simulink model "sefdmConv"  (R2022a)
settings: Solver=VariableStepDiscrete  StartTime=0.0  StopTime=infoBitsPerFrame*100  RelTol=1e-3
InitFcn:
  | run('initSefdmModel.m')
StopFcn:
  | % disp(['ber = ', num2str(out.ber(1))]);
values from neighbouring files (symbols this model uses):
  bitAlloc = ones(N1, 1) * bitsPerSymbol    [initSefdmModel.m]
  bitsPerFrame = dataNum * N1 * bitsPerSymbol    (= 16256)    [initSefdmModel.m]
  codeRate = 1/2    (= 0.5)    [initSefdmModel.m]
  dataNum = 16    [initSefdmModel.m]
  fecLength = 32 / parallelFactor    (= 64)    [initSefdmModel.m]
  fftSize = 512    [initSefdmModel.m]
  infoBitsPerFrame = bitsPerFrame * codeRate - parallel * (constLen - 1)    (= 7366)    [initSefdmModel.m]
  intrlvCol = 1    [initSefdmModel.m]
  intrlvRow = parallel * 2    (= 254)    [initSefdmModel.m]
  N1 = 254    [initSefdmModel.m]
  preamble = preamble(channelInUse, :)    [initSefdmModel.m]
  seed = 42    [initSefdmModel.m]
  symbolsPerFrame = bitsPerFrame / bitsPerSymbol    (= 4064)    [initSefdmModel.m]
  useEqualizer = 1    [initSefdmModel.m]
  useInterleave = 1    [initSefdmModel.m]
  useIteration = 0    [initSefdmModel.m]
libraries: commsink2 x2, dspstat3 x2, commrandsrc3 x1, commchan3 x1, dspindex x1
settings Model: Creator=lsfan  LastModifiedBy=lsfan
settings SolverCC: AlgebraicLoopSolver=TrustRegion
settings DataIOCC: LimitDataPoints=on  SaveOutput=off  SaveTime=off
settings OptimizationCC: BooleanDataType=off  DefaultParameterBehavior=Inlined  LocalBlockOutputs=off  LifeSpan=inf
settings DebuggingCC: AlgebraicLoopMsg=error  SingleTaskRateTransMsg=error  UnconnectedInputMsg=warning  UnconnectedOutputMsg=warning  UnconnectedLineMsg=warning  AllowSymbolicDim=off  SFUnexpectedBacktrackingDiag=warning  SFNoUnconditionalDefaultTransitionDiag=warning  SFExecutionAtInitializationDiag=none  SFMachineParentedDataDiag=warning  ArithmeticOperatorsInVariantConditions=warning
settings SFSimCC: SimUseLocalCustomCode=off  CustomCodeUndefinedFunction=UseInterfaceOnly
settings RTWCC: RTWUseLocalCustomCode=off
settings CodeAppCC: StateflowObjectComments=on
settings GRTTargetCC: TargetLangStandard=C89/C90 (ANSI)
settings ConfigComp: CovMetricSettings=dw  CovSaveCumulativeToWorkspaceVar=on  CovSaveSingleToWorkspaceVar=on  CovExternalEMLEnable=off  CovSFcnEnable=off

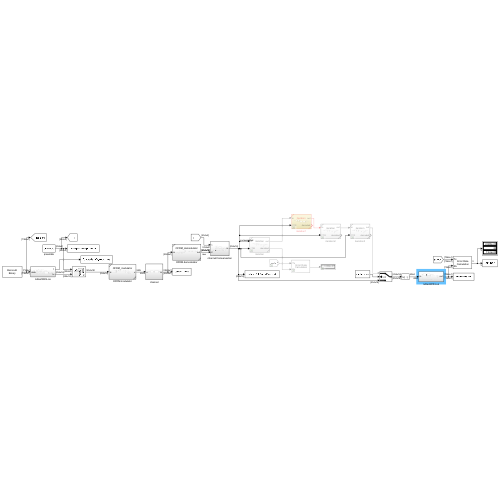
[thumbnail: Simulink's stored preview of the top-level diagram]
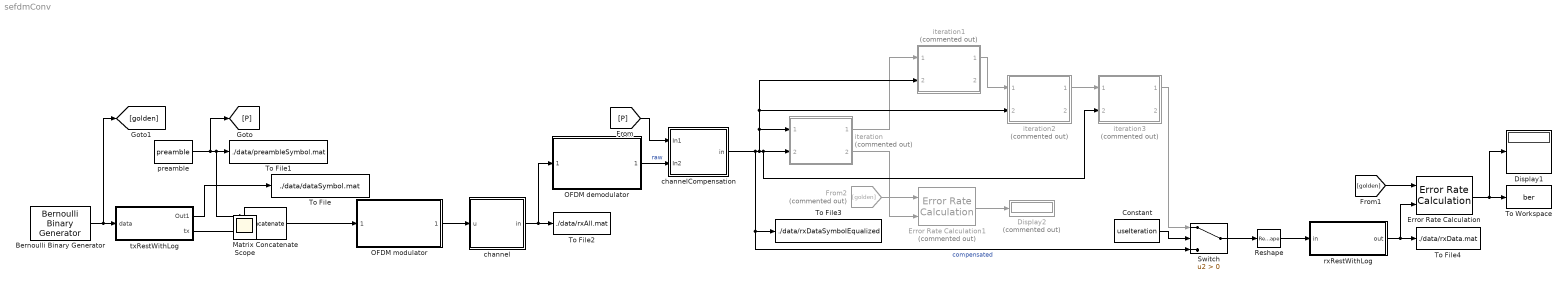
== system sefdmConv ==
  Bernoulli Binary Generator : commrandsrc3/Bernoulli Binary Generator  ProbabilityOfZero=0.5  SeedSource=Parameter  Seed=seed  SampleTime=1  SamplesPerFrame=infoBitsPerFrame  OutputDataType=double  SimulateUsing=Interpreted execution
  Constant : Constant  Value=useIteration
  Display1 : Display
  Display2 : Display  Commented=on
  Error Rate Calculation : commsink2/Error Rate Calculation  N=0  st_delay=0  cp_mode=Entire frame  subframe=[]  PMode=Port  WsName=ErrorVec  RsMode2=off  stop=off  numErr=maxErrNum  maxBits=maxBitsNum
  Error Rate Calculation1 : commsink2/Error Rate Calculation  Commented=on  N=0  st_delay=0  cp_mode=Entire frame  subframe=[]  PMode=Port  WsName=ErrorVec  RsMode2=off  stop=off  numErr=maxErrNum  maxBits=maxBitsNum
  From2 : From  Commented=on  GotoTag=golden
  Matrix Concatenate : Concatenate  Mode=Multidimensional array  ConcatenateDimension=2
  OFDM demodulator : Subsystem  ReferencedSubsystem=OFDM_demodulator
  OFDM modulator : Subsystem  ReferencedSubsystem=OFDM_modulator
  Reshape : Reshape
  Switch : Switch  Criteria=u2 > Threshold  SaturateOnIntegerOverflow=off  InputSameDT=off
  To File : ToFile  Filename=./data/dataSymbol.mat  SaveFormat=Timeseries
  To File1 : ToFile  Filename=./data/preambleSymbol.mat  SaveFormat=Timeseries
  To File2 : ToFile  Filename=./data/rxAll.mat  SaveFormat=Timeseries
  To File3 : ToFile  Filename=./data/rxDataSymbolEqualized  SaveFormat=Timeseries
  To File4 : ToFile  Filename=./data/rxData.mat  SaveFormat=Timeseries
  To Workspace : ToWorkspace  VariableName=ber  SampleTime=-1
      settings: Save2DSignal=2-D array (concatenate along first dimension)
  channel : Subsystem
  channelCompensation : Subsystem
  iteration{,1..3} (4 alike) : Subsystem  Commented=on  ReferencedSubsystem=iteration
  preamble : Constant  Value=preamble
  rxRestWithLog : Subsystem
  txRestWithLog : Subsystem
  Scope : Scope
  wires:
  [golden] -> Error Rate Calculation/1
  iteration2/1 -> iteration3/1
  txRestWithLog/1(Out1) -> To File/1
  txRestWithLog/2(tx) -> Matrix Concatenate/2
  Constant/1 -> Switch/2
  preamble/1 -> Matrix Concatenate/1, To File1/1, [P]
  iteration/1 -> iteration1/1
  From2/1 -> Error Rate Calculation1/1
  OFDM demodulator/1 -> channelCompensation/2(In2)  "raw"
  OFDM modulator/1 -> channel/1(u)
  iteration1/1 -> iteration2/1
  Switch/1 -> Reshape/1
  [P] -> channelCompensation/1(In1)
  Matrix Concatenate/1 -> OFDM modulator/1
  Reshape/1 -> rxRestWithLog/1(in)
  Error Rate Calculation1/1 -> Display2/1
  Bernoulli Binary Generator/1 -> txRestWithLog/1(data), [golden]
  iteration3/1 -> Switch/1
  iteration/2 -> Error Rate Calculation1/2
  Error Rate Calculation/1 -> To Workspace/1, Display1/1
  channel/1(in) -> OFDM demodulator/1, To File2/1
  rxRestWithLog/1(out) -> To File4/1, Error Rate Calculation/2
  channelCompensation/1(in) -> To File3/1, Switch/3, iteration3/2, iteration/2, iteration1/2, iteration2/2, iteration/1  "compensated"

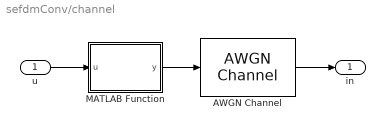
== system sefdmConv/channel ==
  u : Inport
  AWGN Channel : commchan3/AWGN Channel  InputProcessing=Columns as channels (frame based)  seed=67  noiseMode="Signal to noise ratio  (SNR)"  EbNodB=EbNo  EsNodB=10  SNRdB=EbNo  bitsPerSym=bitsPerSymbol  Ps=1 / fftSize  Tsym=bitsPerSymbol  variance=1
  MATLAB Function : MATLAB Function  TreatAsAtomicUnit=on
  in : Outport
  wires:
  MATLAB Function/1(y) -> AWGN Channel/1
  u/1 -> MATLAB Function/1(u)
  AWGN Channel/1 -> in/1

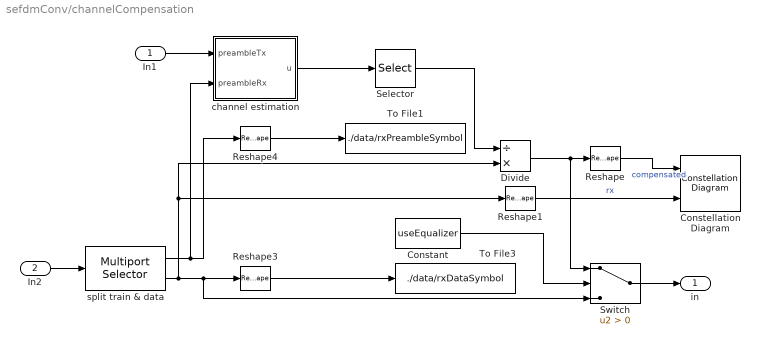
== system sefdmConv/channelCompensation ==
  In1 : Inport
  In2 : Inport  Port=2
  Constant : Constant  Value=useEqualizer
  Constellation Diagram : ConstellationDiagram  NumInputPorts=2  WindowPosition=[2983.000000,244.000000,600.000000,600.000000,]  Visible=on  ScopeFrameLocation=window  ReferenceConstellation="{[16-QAM][0.7071+0.7071i          -0.7071+0.7071i          -0.7071-0.7071i            0.707-0.7071i]}"  ShowLegend=on  DefaultConfigurationName=comm.scopes.ConstellationDiagramBlockCfg
  Divide : Product  Inputs=/*
  Reshape{,1,3..4} (4 alike) : Reshape
  Selector : Selector  NumberOfDimensions=2  InputPortWidth=3  IndexOptions=Select all,Index vector (dialog)  Indices=[1 3],ones(1,dataNum)  OutputSizes=1,1
  Switch : Switch  Criteria=u2 > Threshold  SaturateOnIntegerOverflow=off  InputSameDT=off
  To File1 : ToFile  Filename=./data/rxPreambleSymbol  SaveFormat=Timeseries
  To File3 : ToFile  Filename=./data/rxDataSymbol  SaveFormat=Timeseries
  channel estimation : Subsystem
  split train & data : dspindex/Multiport Selector  rowsOrCols=Columns  idxCellArray={[1:preambleNum], [preambleNum+1:frameNum]}  idxErrMode=Clip Index
  in : Outport
  wires:
  In2/1 -> split train & data/1
  Reshape3/1 -> To File3/1
  Reshape4/1 -> To File1/1
  In1/1 -> channel estimation/1(preambleTx)
  Selector/1 -> Divide/1
  Reshape1/1 -> Constellation Diagram/2  "rx"
  channel estimation/1(u) -> Selector/1
  Constant/1 -> Switch/2
  Switch/1 -> in/1
  Reshape/1 -> Constellation Diagram/1  "compensated"
  Divide/1 -> Switch/1, Reshape/1
  split train & data/2 -> Switch/3, Reshape3/1, Divide/2, Reshape1/1
  split train & data/1 -> channel estimation/2(preambleRx), Reshape4/1

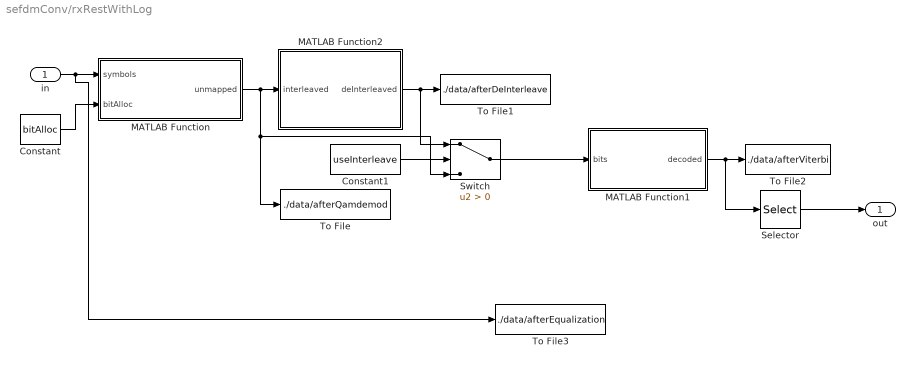
== system sefdmConv/rxRestWithLog ==
  in : Inport
  Constant : Constant  Value=bitAlloc
  Constant1 : Constant  Value=useInterleave
  MATLAB Function : MATLAB Function  TreatAsAtomicUnit=on
  MATLAB Function1 : MATLAB Function  TreatAsAtomicUnit=on
  MATLAB Function2 : MATLAB Function  TreatAsAtomicUnit=on
  Selector : Selector  InputPortWidth=bitsPerFrame * codeRate  IndexOptions=Index vector (dialog)  Indices=[1:infoBitsPerFrame]  OutputSizes=1
  Switch : Switch  Criteria=u2 > Threshold  SaturateOnIntegerOverflow=off  InputSameDT=off
  To File : ToFile  Filename=./data/afterQamdemod  SaveFormat=Timeseries
  To File1 : ToFile  Filename=./data/afterDeInterleave  SaveFormat=Timeseries
  To File2 : ToFile  Filename=./data/afterViterbi  SaveFormat=Timeseries
  To File3 : ToFile  Filename=./data/afterEqualization  SaveFormat=Timeseries
  out : Outport
  wires:
  MATLAB Function1/1(decoded) -> To File2/1, Selector/1
  Constant1/1 -> Switch/2
  MATLAB Function/1(unmapped) -> Switch/3, To File/1, MATLAB Function2/1(interleaved)
  Constant/1 -> MATLAB Function/2(bitAlloc)
  Switch/1 -> MATLAB Function1/1(bits)
  Selector/1 -> out/1
  in/1 -> To File3/1, MATLAB Function/1(symbols)
  MATLAB Function2/1(deInterleaved) -> To File1/1, Switch/1

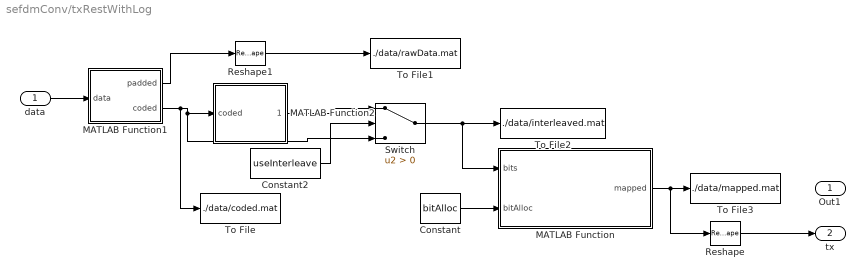
== system sefdmConv/txRestWithLog ==
  data : Inport
  Constant : Constant  Value=bitAlloc
  Constant2 : Constant  Value=useInterleave
  MATLAB Function : MATLAB Function  TreatAsAtomicUnit=on
  MATLAB Function1 : MATLAB Function  TreatAsAtomicUnit=on
  MATLAB Function2 : MATLAB Function  TreatAsAtomicUnit=on
  Reshape : Reshape  OutputDimensionality=Customize  OutputDimensions=[N1, symbolsPerFrame / N1]
  Reshape1 : Reshape
  Switch : Switch  Criteria=u2 > Threshold  SaturateOnIntegerOverflow=off  InputSameDT=off
  To File : ToFile  Filename=./data/coded.mat  SaveFormat=Timeseries
  To File1 : ToFile  Filename=./data/rawData.mat  SaveFormat=Timeseries
  To File2 : ToFile  Filename=./data/interleaved.mat  SaveFormat=Timeseries
  To File3 : ToFile  Filename=./data/mapped.mat  SaveFormat=Timeseries
  Out1 : Outport
  tx : Outport  Port=2
  wires:
  MATLAB Function2/1(interleaved) -> Switch/1
  Constant/1 -> MATLAB Function/2(bitAlloc)
  Switch/1 -> MATLAB Function/1(bits), To File2/1
  Reshape1/1 -> To File1/1
  MATLAB Function1/2(coded) -> Switch/3, MATLAB Function2/1(coded), To File/1
  data/1 -> MATLAB Function1/1(data)
  MATLAB Function/1(mapped) -> Reshape/1, To File3/1
  Reshape/1 -> tx/1
  MATLAB Function1/1(padded) -> Reshape1/1
  Constant2/1 -> Switch/2

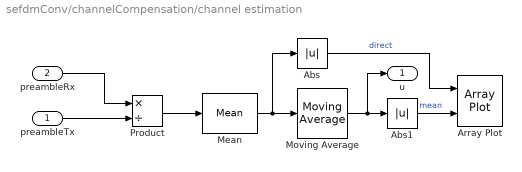
== system sefdmConv/channelCompensation/channel estimation ==
  preambleTx : Inport
  preambleRx : Inport  Port=2
  Abs : Abs  SaturateOnIntegerOverflow=off
  Abs1 : Abs  SaturateOnIntegerOverflow=off
  Array Plot : ArrayPlot  NumInputPorts=2  WindowPosition=[3842.000000,45.000000,1278.000000,1360.000000,]  Visible=on  ScopeFrameLocation=window  YLimits=[-0.0556,2.4257]  ShowLegend=on
  Mean : dspstat3/Mean  run=off  InputProcessing=Columns as channels (frame based)  reset_popup=None  directionMode=Each row  dimension=1  roiEnable=off  roiType=Rectangles  roiPortion=Entire ROI  roiOutput=Individual statistics for each ROI  roiFlag=off  roundingMode=Floor  overflowMode=off  outputDataTypeStr=Inherit: Same as accumulator  outputMin=[]  outputMax=[]  outputLastDataTypeStr=Inherit: Same as accumulator
  Moving Average : dspstat3/Moving Average  Method=Sliding window  ForgettingFactorPort=off  SpecifyWindowLength=on  WindowLength=movingAvgLength  ForgettingFactor=0.9  SimulateUsing=Code generation
  Product : Product  Inputs=*/
  u : Outport
  wires:
  Product/1 -> Mean/1
  preambleTx/1 -> Product/2
  Moving Average/1 -> Abs1/1, u/1
  preambleRx/1 -> Product/1
  Abs/1 -> Array Plot/1  "direct"
  Mean/1 -> Moving Average/1, Abs/1
  Abs1/1 -> Array Plot/2  "mean"

== matlab function sefdmConv/channel/MATLAB Function ==
  data: u input; y output
function y = channelFilter(u)
    y = filter([1, 0.8, 0.1, 0.05, 0.01, 0.005], 1, u);

== matlab function sefdmConv/rxRestWithLog/MATLAB Function ==
  data: symbols input; unmapped output; bitAlloc input; N1 parameter
function unmapped = qamdemodFtn(symbols, bitAlloc, N1)
    
    matrix = reshape(symbols, numel(bitAlloc), []);

    temp = zeros(N1 * 4, 16);
    
    current = 0;
    row = 1;
    
    for i = 1:N1
        bit = bitAlloc(i);
        slice = matrix(row, :);
        temp(current+1:current+bit, :) = qamdemod(slice, 2^bit, 'OutputType', 'bit', 'UnitAveragePower', 1);
        current = current + bit;
        row = row + 1;
    end

    unmapped = reshape(temp, [], 1);
    
end

== matlab function sefdmConv/rxRestWithLog/MATLAB Function1 ==
  data: bits input; decoded output; fecLength parameter; parallel parameter
function decoded = vitdecFTN(bits, fecLength, parallel)

    trellis = poly2trellis(7, [171,133]);
    bits = reshape(bits, parallel, []);
    temp = zeros(parallel,fecLength);
    
    for i = 1:parallel
        slice = bits(i, :);
        temp(i,:) = vitdec(slice, trellis, fecLength,'term', 'hard');
    end

    decoded = reshape(temp, [], 1);
end

== matlab function sefdmConv/rxRestWithLog/MATLAB Function2 ==
  data: interleaved input; deInterleaved output; parallel parameter; intrlvCol parameter; intrlvRow parameter
function deInterleaved = deInterleave(interleaved, parallel, intrlvCol, intrlvRow)

    interleaved = reshape(interleaved, parallel * 2, 64);
    container = zeros(parallel * 2, 64);
    for i = 1:64
        column = interleaved(:,i);
        temp = circshift(column, -i*4);  % spatial permutation
        container(:, i) = matintrlv(temp, intrlvCol, intrlvRow);; % spatial permutation by circular shift
    end

    deInterleaved = reshape(container, [], 1);

== matlab function sefdmConv/txRestWithLog/MATLAB Function ==
  data: bits input; mapped output; bitAlloc input; N1 parameter
function mapped = qammodFtn(bits, bitAlloc, N1)
    matrix = reshape(bits, sum(bitAlloc), []);

    temp = complex(zeros(N1, 16));
    
    current = 0;
    row = 1;
    
    for i = 1:N1
        bit = bitAlloc(i);
        slice = matrix(current + 1: current + bit, :);
        temp(row, :) = qammod(slice, 2^bit, 'InputType', 'bit', 'UnitAveragePower', 1);
        current = current + bit;
        row = row + 1;
    end

    mapped = reshape(temp, [], 1);
    
end

== matlab function sefdmConv/txRestWithLog/MATLAB Function1 ==
  data: padded output; data input; coded output; parallel parameter; fecLength parameter
function [padded, coded] = convencFTN(data, parallel, fecLength)
    
    trellis = poly2trellis(7, [171,133]);
    data = reshape(data, parallel, fecLength-6);
    padded = [data, zeros(parallel, 6)]; % padding 0s
    
    temp = zeros(parallel,fecLength*2);
    for i = 1:parallel
        slice = padded(i, :);
        temp(i,:) = convenc(slice, trellis);
    end

    coded = reshape(temp, [], 1);
end

== matlab function sefdmConv/txRestWithLog/MATLAB Function2 ==
  data: coded input; interleaved output; parallel parameter; intrlvRow parameter; intrlvCol parameter
function interleaved = interleave(coded, parallel, intrlvRow, intrlvCol)

    coded = reshape(coded, parallel * 2, 64);
    container = zeros(parallel * 2, 64);
    for i = 1:64
        column = coded(:,i);
        temp = matintrlv(column, intrlvRow, intrlvCol); % spatial permutation
        container(:, i) = circshift(temp, i*4); % spatial permutation by circular shift
    end

    interleaved = reshape(container, [], 1);
